simulink model "simulation"  (R2024b)
settings: Solver=FixedStepAuto  StartTime=0.0  StopTime=15  FixedStep=0.01  RelTol=1e-3
undefined symbols (not defined in the file or in its folder): magnitude, rate, servo_latency
libraries: aerolibatmos2 x1, aerolibasang x1, shared6dof x1, aerolibanim x1, aerolibnav x1
settings Model: Creator=Sebastian Bagley  LastModifiedBy=Sebastian Bagley

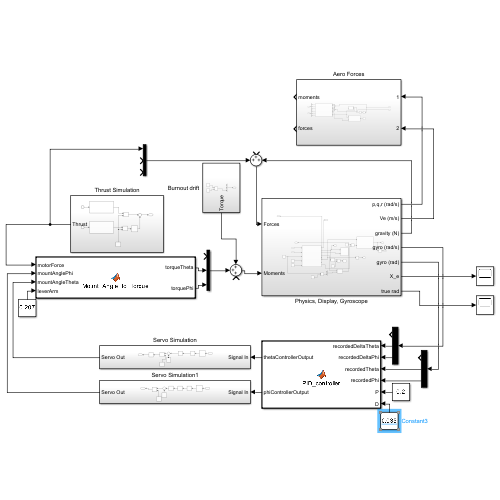
[thumbnail: Simulink's stored preview of the top-level diagram]
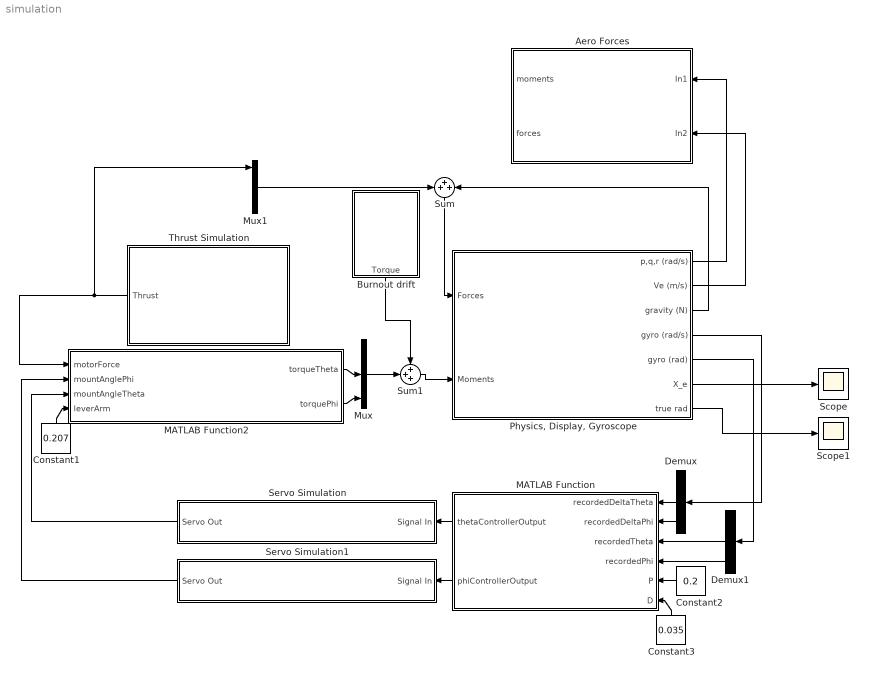
== system simulation ==
  Aero Forces : Subsystem
  Burnout drift : Subsystem
  Constant1 : Constant  Value=0.207
  Constant2 : Constant  Value=0.2
  Constant3 : Constant  Value=0.035
  Demux : Demux  Outputs=3
  Demux1 : Demux  Outputs=3
  MATLAB Function : MATLAB Function  TreatAsAtomicUnit=on
  MATLAB Function2 : MATLAB Function  TreatAsAtomicUnit=on
  Mux : Mux  Inputs=3
  Mux1 : Mux  Inputs=3
  "Physics, Display, Gyroscope" : Subsystem
  Scope : Scope
  Scope1 : Scope
  Servo Simulation : Subsystem
  Servo Simulation1 : Subsystem
  Sum : Sum  Inputs=+++
  Sum1 : Sum  Inputs=+++
  Thrust Simulation : Subsystem
  wires:
  Constant1/1 -> MATLAB Function2/4(leverArm)
  Constant3/1 -> MATLAB Function/6(D)
  Demux/2 -> MATLAB Function/1(recordedDeltaTheta)
  Demux/3 -> MATLAB Function/2(recordedDeltaPhi)
  Demux1/3 -> MATLAB Function/4(recordedPhi)
  Demux1/2 -> MATLAB Function/3(recordedTheta)
  Mux1/1 -> Sum/1
  MATLAB Function2/1(torqueTheta) -> Mux/2
  MATLAB Function2/2(torquePhi) -> Mux/3
  "Physics, Display, Gyroscope"/1(p,q,r (rad/s)) -> Aero Forces/1(In1)
  "Physics, Display, Gyroscope"/2(Ve (m/s)) -> Aero Forces/2(In2)
  "Physics, Display, Gyroscope"/5(gyro (rad)) -> Demux1/1
  "Physics, Display, Gyroscope"/4(gyro (rad/s)) -> Demux/1
  "Physics, Display, Gyroscope"/3(gravity (N)) -> Sum/3
  Mux/1 -> Sum1/2
  MATLAB Function/1(thetaControllerOutput) -> Servo Simulation/1(Signal In)
  MATLAB Function/2(phiControllerOutput) -> Servo Simulation1/1(Signal In)
  Servo Simulation/1(Servo Out) -> MATLAB Function2/3(mountAngleTheta)
  Servo Simulation1/1(Servo Out) -> MATLAB Function2/2(mountAnglePhi)
  Constant2/1 -> MATLAB Function/5(P)
  Sum1/1 -> "Physics, Display, Gyroscope"/2(Moments)
  Sum/1 -> "Physics, Display, Gyroscope"/1(Forces)
  Thrust Simulation/1(Thrust) -> Mux1/1, MATLAB Function2/1(motorForce)
  Burnout drift/1(Torque) -> Sum1/1
  "Physics, Display, Gyroscope"/6(X_e) -> Scope/1
  "Physics, Display, Gyroscope"/7(true rad) -> Scope1/1

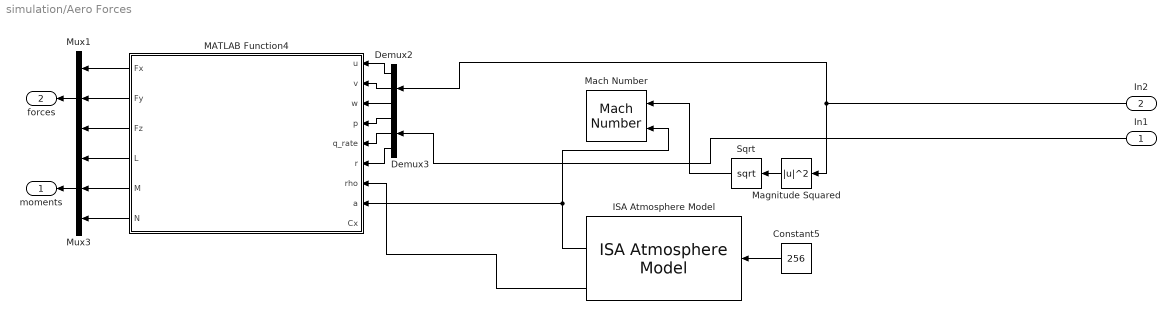
== system simulation/Aero Forces ==
  In1 : Inport
  In2 : Inport  Port=2
  Constant5 : Constant  Value=256
  Demux2 : Demux  Outputs=3
  Demux3 : Demux  Outputs=3
  ISA Atmosphere Model : aerolibatmos2/ISA Atmosphere Model  useExtended=off  action=Warning  custom=off  viscosityOut=off  g=9.80665  gamma=1.4  R=287.0531  L=0.0065  h_trop=11000  h_strat=20000  rho0=1.225  P0=101325  T0=288.15  h0=0  S=110.4  Tref=273.15  muref=1.716e-5
  MATLAB Function4 : MATLAB Function  TreatAsAtomicUnit=on
  Mach Number : aerolibasang/Mach Number
  Magnitude Squared : Math  Operator=magnitude^2
  Mux1 : Mux  Inputs=3
  Mux3 : Mux  Inputs=3
  Sqrt : Sqrt
  moments : Outport
  forces : Outport  Port=2
  wires:
  Demux3/2 -> MATLAB Function4/5(q_rate)
  In1/1 -> Demux3/1
  Demux2/1 -> MATLAB Function4/1(u)
  ISA Atmosphere Model/2 -> MATLAB Function4/8(a), Mach Number/2
  Demux3/1 -> MATLAB Function4/4(p)
  ISA Atmosphere Model/4 -> MATLAB Function4/7(rho)
  Sqrt/1 -> Mach Number/1
  MATLAB Function4/4(L) -> Mux3/1
  Demux3/3 -> MATLAB Function4/6(r)
  Magnitude Squared/1 -> Sqrt/1
  MATLAB Function4/6(N) -> Mux3/3
  MATLAB Function4/5(M) -> Mux3/2
  In2/1 -> Magnitude Squared/1, Demux2/1
  Constant5/1 -> ISA Atmosphere Model/1
  Demux2/3 -> MATLAB Function4/3(w)
  Mux3/1 -> moments/1
  Demux2/2 -> MATLAB Function4/2(v)
  Mux1/1 -> forces/1
  MATLAB Function4/2(Fy) -> Mux1/2
  MATLAB Function4/3(Fz) -> Mux1/3
  MATLAB Function4/1(Fx) -> Mux1/1

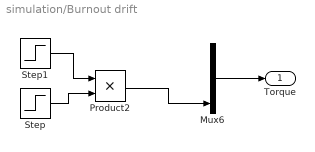
== system simulation/Burnout drift ==
  Mux6 : Mux  Inputs=3
  Product2 : Product
  Step : Step  Time=2.9  After=0.075  SampleTime=0
  Step1 : Step  Time=3.2  Before=1  After=0  SampleTime=0
  Torque : Outport
  wires:
  Step/1 -> Product2/2
  Step1/1 -> Product2/1
  Product2/1 -> Mux6/3
  Mux6/1 -> Torque/1

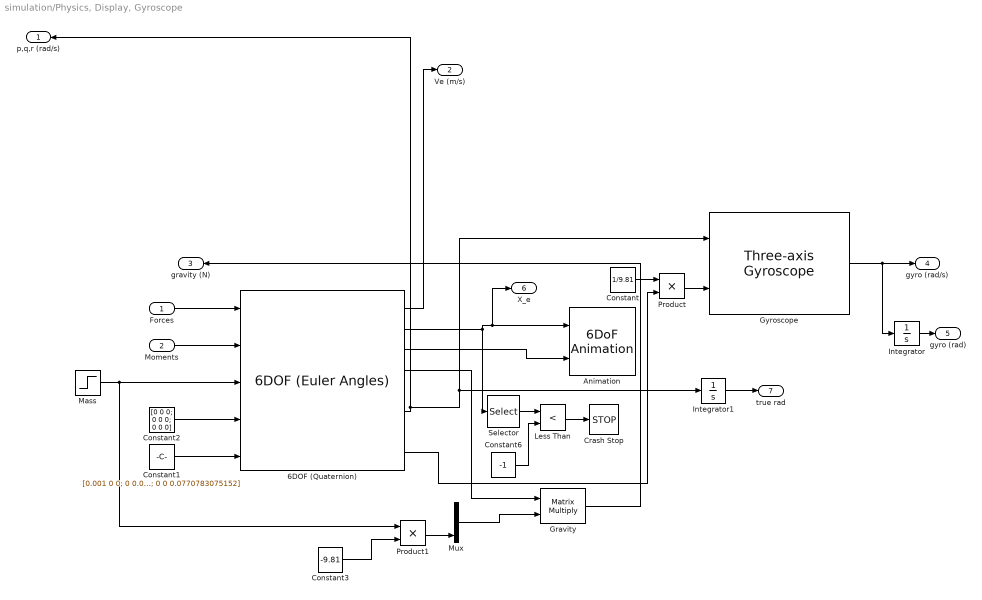
== system simulation/Physics, Display, Gyroscope ==
  Forces : Inport
  Moments : Inport  Port=2
  6DOF (Quaternion) : shared6dof/6DOF (Euler Angles)  units=Metric (MKS)  mtype=Custom Variable  rep=Quaternion  xme_0=[0 0 0]  Vm_0=[0 0 0]  eul_0=[0 -3.14159/2 0]  pm_0=[0 0 0]  mass_0=1.7  mass_e=0.5  mass_f=2.0  inertia=[0.001 0 0; 0 0.0770783075152 0; 0 0 0.0770783075152]  inertia_e=eye(3)  inertia_f=2*eye(3)  k_quat=1.0  vre_flag=off  abi_flag=off  aMode=0  xme_statename=''  Vm_statename=''  eul_statename=''  quat_statename=''  pm_statename=''  mass_statename=''
      settings: LibrarySourceBlock=aerolib6dof2/6DOF (Quaternion)
  Animation : aerolibanim/6DoF Animation  u1=[0 4000 -2000 2000 -5000 -3000]  u2=0.01  u3=3  u4=[4000 0 -5000]  u5=Fixed position  u6=[-50 0 0]  u7=10  u8=on
  Constant : Constant  Value=1/9.81
  Constant1 : Constant  Value=[0.001 0 0; 0 0.0770783075152 0; 0 0 0.0770783075152]
  Constant2 : Constant  Value=[0 0 0; 0 0 0; 0 0 0]
  Constant3 : Constant  Value=-9.81
  Constant6 : Constant  Value=-1
  Crash Stop : Stop
  Gravity : Product  Multiplication=Matrix(*)
  Gyroscope : aerolibnav/Three-axis Gyroscope  dtype_g=on  w_g=190  z_g=0.707  g_sf_cc=[1 0 0; 0 1 0; 0 0 1]  g_bias=[0 0 0]  g_sen=[0 0 0]  g_Ts=0  g_rand=on  g_seeds=[23093 23094 23095]  g_pow=[0.000001 0.000001 0.000001]  g_sat="[-inf  -inf  -inf  inf inf inf]"
  Integrator : Integrator
  Integrator1 : Integrator
  Less Than : RelationalOperator  Operator=<  OutDataTypeStr=boolean  RndMeth=Simplest  InputSameDT=off
  Mass : Step  Time=3.4  Before=1.963  After=1.963-0.09  SampleTime=0
  Mux : Mux  Inputs=3
  Product : Product
  Product1 : Product
  Selector : Selector  InputPortWidth=3  IndexOptions=Index vector (dialog)  Indices=[3]  OutputSizes=1
  p,q,r (rad/s) : Outport
  Ve (m/s) : Outport  Port=2
  gravity (N) : Outport  Port=3
  gyro (rad/s) : Outport  Port=4
  gyro (rad) : Outport  Port=5
  X_e : Outport  Port=6
  true rad : Outport  Port=7
  wires:
  6DOF (Quaternion)/3 -> Animation/2
  Forces/1 -> 6DOF (Quaternion)/1
  6DOF (Quaternion)/2 -> X_e/1, Animation/1, Selector/1
  Selector/1 -> Less Than/1
  6DOF (Quaternion)/6 -> p,q,r (rad/s)/1, Integrator1/1, Gyroscope/1
  Gyroscope/1 -> Integrator/1, gyro (rad/s)/1
  Constant/1 -> Product/1
  6DOF (Quaternion)/4 -> Gravity/1
  6DOF (Quaternion)/8 -> Product/2
  Product/1 -> Gyroscope/2
  Moments/1 -> 6DOF (Quaternion)/2
  Less Than/1 -> Crash Stop/1
  Constant6/1 -> Less Than/2
  6DOF (Quaternion)/1 -> Ve (m/s)/1
  Gravity/1 -> gravity (N)/1
  Integrator/1 -> gyro (rad)/1
  Integrator1/1 -> true rad/1
  Constant2/1 -> 6DOF (Quaternion)/4
  Constant1/1 -> 6DOF (Quaternion)/5
  Mass/1 -> Product1/1, 6DOF (Quaternion)/3
  Product1/1 -> Mux/3
  Constant3/1 -> Product1/2
  Mux/1 -> Gravity/2

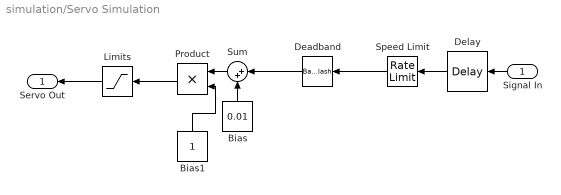
== system simulation/Servo Simulation ==
  Signal In : Inport
  Bias : Constant  Value=0.01
  Bias1 : Constant
  Deadband : Backlash  BacklashWidth=backlash
  Delay : TransportDelay  DelayTime=servo_latency
  Limits : Saturate  UpperLimit=0.0872665  LowerLimit=-0.0872665
  Product : Product
  Speed Limit : RateLimiter  RisingSlewLimit=rate  FallingSlewLimit=-rate  SampleTimeMode=inherited
  Sum : Sum  Inputs=|++
  Servo Out : Outport
  wires:
  Delay/1 -> Speed Limit/1
  Signal In/1 -> Delay/1
  Deadband/1 -> Sum/1
  Bias/1 -> Sum/2
  Sum/1 -> Product/1
  Bias1/1 -> Product/2
  Speed Limit/1 -> Deadband/1
  Product/1 -> Limits/1
  Limits/1 -> Servo Out/1

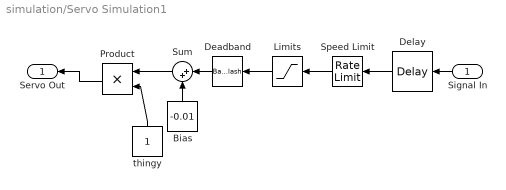
== system simulation/Servo Simulation1 ==
  Signal In : Inport
  Bias : Constant  Value=-0.01
  Deadband : Backlash  BacklashWidth=backlash
  Delay : TransportDelay  DelayTime=servo_latency
  Limits : Saturate  UpperLimit=0.0872665  LowerLimit=-0.0872665
  Product : Product
  Speed Limit : RateLimiter  RisingSlewLimit=rate  FallingSlewLimit=-rate  SampleTimeMode=inherited
  Sum : Sum  Inputs=|++
  thingy : Constant
  Servo Out : Outport
  wires:
  Limits/1 -> Deadband/1
  Delay/1 -> Speed Limit/1
  Speed Limit/1 -> Limits/1
  Signal In/1 -> Delay/1
  Deadband/1 -> Sum/1
  Bias/1 -> Sum/2
  Sum/1 -> Product/1
  Product/1 -> Servo Out/1
  thingy/1 -> Product/2

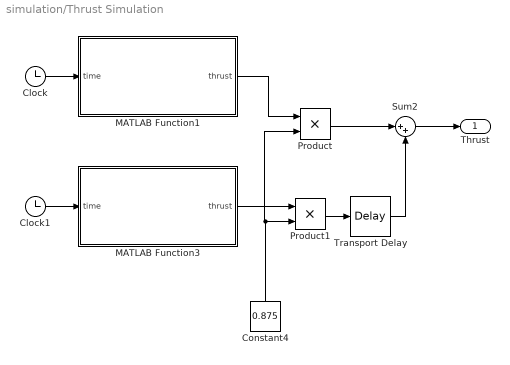
== system simulation/Thrust Simulation ==
  Clock : Clock
  Clock1 : Clock
  Constant4 : Constant  Value=0.875
  MATLAB Function1 : MATLAB Function  TreatAsAtomicUnit=on
  MATLAB Function3 : MATLAB Function  TreatAsAtomicUnit=on
  Product : Product
  Product1 : Product
  Sum2 : Sum  Inputs=|++
  Transport Delay : TransportDelay  DelayTime=4.7
  Thrust : Outport
  wires:
  Clock1/1 -> MATLAB Function3/1(time)
  Product/1 -> Sum2/1
  Transport Delay/1 -> Sum2/2
  Clock/1 -> MATLAB Function1/1(time)
  Constant4/1 -> Product/2, Product1/2
  Product1/1 -> Transport Delay/1
  MATLAB Function1/1(thrust) -> Product/1
  MATLAB Function3/1(thrust) -> Product1/1
  Sum2/1 -> Thrust/1

== matlab function simulation/Thrust Simulation/MATLAB Function1 ==
  settings: updateMethod=DISCRETE
  data: thrust output; time input
function thrust = Motor_Simulation(time)
% Returns thrust in newtons for given time in seconds by interpolating the
% engine thrust curve
    persistent t_data f_data initialized;

    % Load the engine data
    if isempty(initialized)
        engine_data = {
            '<eng-data cg="49." f="0." m="38.8" t="0."/>';
            '<eng-data cg="49." f="57.631" m="38.1838" t="0.039"/>';
            '<eng-data cg="49." f="53.491" m="33.6753" t="0.187"/>';
            '<eng-data cg="49." f="51.239" m="29.2252" t="0.342"/>';
            '<eng-data cg="49." f="47.86" m="24.9328" t="0.5"/>';
            '<eng-data cg="49." f="33.806" m="13.7388" t="1."/>';
            '<eng-data cg="49." f="22.94" m="5.96068" t="1.5"/>';
            '<eng-data cg="49." f="10.135" m="1.42709" t="2."/>';
            '<eng-data cg="49." f="4.504" m="0.596372" t="2.207"/>';
            '<eng-data cg="49." f="0." m="0." t="2.69"/>';
        };

        N = numel(engine_data);
        t_raw = zeros(N, 1);
        f_raw = zeros(N, 1);

        % Get the time and thrust values
        for k = 1:N
            s = engine_data{k};
            
            % Find and extract time
            t_pattern_start = 't="';
            idx_t_pattern_start = strfind(s, t_pattern_start);
            idx_t_value_start = idx_t_pattern_start(1) + length(t_pattern_start);
            idx_t_value_end_relative = strfind(s(idx_t_value_start:end), '"');
            idx_t_value_end = idx_t_value_start + idx_t_value_end_relative(1) - 2;
            t_str = s(idx_t_value_start : idx_t_value_end);
            t_raw(k) = real(str2double(t_str));

            % Find and extract force
            f_pattern_start = 'f="';
            idx_f_pattern_start = strfind(s, f_pattern_start);
            idx_f_value_start = idx_f_pattern_start(1) + length(f_pattern_start);
            idx_f_value_end_relative = strfind(s(idx_f_value_start:end), '"');
            idx_f_value_end = idx_f_value_start + idx_f_value_end_relative(1) - 2;
            f_str = s(idx_f_value_start : idx_f_value_end);
            f_raw(k) = real(str2double(f_str));
        end

        % Sort data by time
        [t_sorted, sort_idx] = sort(t_raw);
        f_sorted = f_raw(sort_idx);

        % handle any duplicates
        [t_unique, unique_idx] = unique(t_sorted, 'last');
        
        % store everything in the persistent variable
        t_data = t_unique;
        f_data = f_sorted(unique_idx);

        initialized = true;
    end

    % get the thrust each step from initialization
    thrust = interp1(t_data, f_data, time, 'linear', 0);

end

== matlab function simulation/MATLAB Function ==
  data: recordedDeltaTheta input; thetaControllerOutput output; recordedDeltaPhi input; recordedTheta input; recordedPhi input; P input; D input; phiControllerOutput output
function [thetaControllerOutput,phiControllerOutput]= PD_controller(recordedDeltaTheta,recordedDeltaPhi, recordedTheta, recordedPhi, P, D)
thetaControllerOutput = -P * recordedTheta - D * recordedDeltaTheta;
phiControllerOutput = -P * recordedPhi - D * recordedDeltaPhi;
end

== matlab function simulation/MATLAB Function2 ==
  data: motorForce input; torqueTheta output; mountAnglePhi input; mountAngleTheta input; leverArm input; torquePhi output
function [torqueTheta, torquePhi] = Mount_Angle_to_Torque(motorForce, mountAnglePhi, mountAngleTheta,leverArm)
    torqueTheta = motorForce * leverArm * sin(mountAngleTheta);
    torquePhi = motorForce * leverArm * sin(mountAnglePhi);
end

== matlab function simulation/Thrust Simulation/MATLAB Function3 ==
  settings: updateMethod=DISCRETE
  data: thrust output; time input
function thrust = Motor_Simulation(time)
% Motor_Simulation  Return thrust [N] for given time(s) [s] by
%                   interpolating the engine thrust curve.
%
% This function is fully compatible with Simulink code generation. It uses
% robust strfind parsing and correctly handles duplicate time points.

    % Declare persistent variables to store the processed thrust curve.
    persistent t_data f_data initialized;

    % --- Initialization (runs only once at the start of simulation) ---
    if isempty(initialized)
        engine_data = {
            '<eng-data cg="49." f="0." m="38.8" t="0."/>';
            '<eng-data cg="49." f="57.631" m="38.1838" t="0.039"/>';
            '<eng-data cg="49." f="53.491" m="33.6753" t="0.187"/>';
            '<eng-data cg="49." f="51.239" m="29.2252" t="0.342"/>';
            '<eng-data cg="49." f="47.86" m="24.9328" t="0.5"/>';
            '<eng-data cg="49." f="33.806" m="13.7388" t="1."/>';
            '<eng-data cg="49." f="22.94" m="5.96068" t="1.5"/>';
            '<eng-data cg="49." f="10.135" m="1.42709" t="2."/>';
            '<eng-data cg="49." f="4.504" m="0.596372" t="2.207"/>';
            '<eng-data cg="49." f="0." m="0." t="2.69"/>';
        };

        N = numel(engine_data);
        t_raw = zeros(N, 1);
        f_raw = zeros(N, 1);

        % --- Extract t and f values using Coder-Compatible strfind ---
        for k = 1:N
            s = engine_data{k};
            
            % Find and extract 't' value
            t_pattern_start = 't="';
            idx_t_pattern_start = strfind(s, t_pattern_start);
            idx_t_value_start = idx_t_pattern_start(1) + length(t_pattern_start);
            idx_t_value_end_relative = strfind(s(idx_t_value_start:end), '"');
            idx_t_value_end = idx_t_value_start + idx_t_value_end_relative(1) - 2;
            t_str = s(idx_t_value_start : idx_t_value_end);
            % FIX: Explicitly take the real part to satisfy the Coder
            t_raw(k) = real(str2double(t_str));

            % Find and extract 'f' value
            f_pattern_start = 'f="';
            idx_f_pattern_start = strfind(s, f_pattern_start);
            idx_f_value_start = idx_f_pattern_start(1) + length(f_pattern_start);
            idx_f_value_end_relative = strfind(s(idx_f_value_start:end), '"');
            idx_f_value_end = idx_f_value_start + idx_f_value_end_relative(1) - 2;
            f_str = s(idx_f_value_start : idx_f_value_end);
            % FIX: Explicitly take the real part to satisfy the Coder
            f_raw(k) = real(str2double(f_str));
        end

        % Sort data by time to ensure it's monotonically increasing
        [t_sorted, sort_idx] = sort(t_raw);
        f_sorted = f_raw(sort_idx);

        % --- Handle Duplicate Time Points ---
        [t_unique, unique_idx] = unique(t_sorted, 'last');
        
        % Store the final, clean data in persistent variables
        t_data = t_unique;
        f_data = f_sorted(unique_idx);

        % Mark initialization as complete
        initialized = true;
    end % --- End of Initialization ---

    % --- Runtime Execution (runs at each simulation step) ---
    thrust = interp1(t_data, f_data, time, 'linear', 0);

end

== matlab function simulation/Aero Forces/MATLAB Function4 ==
  data: u input; Fx output; v input; w input; p input; q_rate input; r input; rho input; a input; Cx input; Fy output; Fz output; L output; M output; N output
function [Fx,Fy,Fz,L,M,N] = AeroForcesAndMoments(u,v,w,p,q_rate,r,rho,a,Cx)
% u,v,w    : body translational velocities [m/s]
% p,q_rate,r : body rates [rad/s]
% rho,a    : air density [kg/m^3], speed of sound [m/s]
% Cx       : axial coefficient (≈ Cd at small AoA) from your lookup
% params   : struct with fields (set once in workspace or mask):
%   Sref   [m^2]  reference area (pi*(D/2)^2)
%   Lref   [m]    reference length (overall length)
%   CNa    [1/rad] total normal-force slope
%   CYb    [1/rad] (optional) sideforce slope vs beta; default = 0.8*CNa
%   Cm_a   [1/rad] (optional) pitch-moment slope vs alpha.
%                 If omitted but xcp,xcg given, we compute Cm_a = -CNa*(xcp-xcg)/Lref
%   xcp    [m]     (optional) CP from nose tip
%   xcg    [m]     (optional) CG from nose tip
%   Cmq    [-]     (optional) pitch-rate damping; default = -20
%   Clp    [-]     (optional) roll-rate damping; default = 0
%   Cnr    [-]     (optional) yaw-rate damping;  default = 0
%
% Outputs: body-axis forces [N] and moments [N*m] about CG.

params = struct;
params.Sref = pi*(0.07874/2)^2;      % example: 89 mm OD
params.Lref = 0.8128;                % example: 95 cm long
params.CNa  = 1.908;                 % from OpenRocket (per rad)
params.xcp  = 0.176;                % m from nose (OR readout)
params.xcg  = 0.6096;                % m from nose (your mass model)
params.CYb  = 0.8*1.908;      % decent first guess
params.Cmq  = -22;                 % pitch-rate damping
params.Clp  = 0;                   % roll damping (set if you model roll)
params.Cnr  = 0;                   % yaw damping

% --- Speeds / angles ---
V = sqrt(max(u*u + v*v + w*w, 1e-9));
qbar = 0.5*rho*V*V;                     % dynamic pressure
Mach = V / max(a,1e-6);                 %#ok<NASGU> kept for debugging if you want to output it

% Standard body-axis angle definitions (x fwd, z down)
alpha = atan2(-w, max(u,1e-9));         % +alpha = nose up
sb = max(-1,min(1, v/max(V,1e-9)));     % clamp for asin
beta  = asin(sb);                        % +beta  = wind from right

% --- Coefficient models ---
CNa   = params.CNa;
CYb   = iff(isfield(params,'CYb'), params.CYb, 0.8*CNa);
Cm_a  = get_Cm_a(params, CNa);

Cmq   = iff(isfield(params,'Cmq'), params.Cmq, -20);
Clp   = iff(isfield(params,'Clp'), 0+params.Clp, 0);
Cnr   = iff(isfield(params,'Cnr'), 0+params.Cnr, 0);

% Small-angle linearized normal/side coefficients
CZ = CNa * alpha;                        % +Z (down) for +alpha
CY = CYb * beta;                         % +Y (right) for +beta

% Pitching moment (about CG), with rate damping
Cm = Cm_a*alpha + Cmq * ( q_rate * params.Lref / max(2*V,1e-9) );

% Simple roll/yaw damping (optional; zeros by default)
Cl = Clp * ( p * params.Lref / max(2*V,1e-9) );
Cn = Cnr * ( r * params.Lref / max(2*V,1e-9) );

% --- Convert coefficients to forces/moments in BODY axes ---
% Resolve axial/normal through alpha so X/Z behave correctly as alpha grows
S = params.Sref;  Lref = params.Lref;

X = -qbar*S * ( Cx*cos(alpha) - CZ*sin(alpha) );  % forward (+X) positive
Z =  qbar*S * ( Cx*sin(alpha) + CZ*cos(alpha) );  % down (+Z) positive
Y =  qbar*S * CY;                                 % right (+Y) positive

L = qbar*S*Lref * Cl;                             % roll  about +X
M = qbar*S*Lref * Cm;                             % pitch about +Y
N = qbar*S*Lref * Cn;                             % yaw   about +Z

Fx = X; Fy = Y; Fz = Z;

% ---- helpers ----
function out = iff(tf, a, b)
  if tf, out = a; else, out = b; end
end

function Cm_a = get_Cm_a(p, CNa)
  if isfield(p,'Cm_a')
     Cm_a = p.Cm_a;
  elseif isfield(p,'xcp') && isfield(p,'xcg') && isfield(p,'Lref')
     Cm_a = -CNa * (p.xcp - p.xcg) / p.Lref;
  else
     Cm_a = 0;   % fallback; set explicitly if you see neutral/unstable behavior not intended
  end
end
end
